simulink model "proyecto_simulink"  (R2023b)
settings: Solver=VariableStepAuto  StartTime=0.0  StopTime=0.1  RelTol=1e-3
undefined symbols (not defined in the file): test_ac1, test_ac2, test_ac3, test_am1, test_am2, test_am3, test_fc1, test_fc1_receptor, test_fc2, test_fc2_receptor, test_fc3, test_fc3_receptor, test_fm1, test_fm2, test_fm3, test_mu, test_noise_factor, test_ts
libraries: commanapbnd3 x4
settings Model: Creator=RomaW11  LastModifiedBy=RomaW11

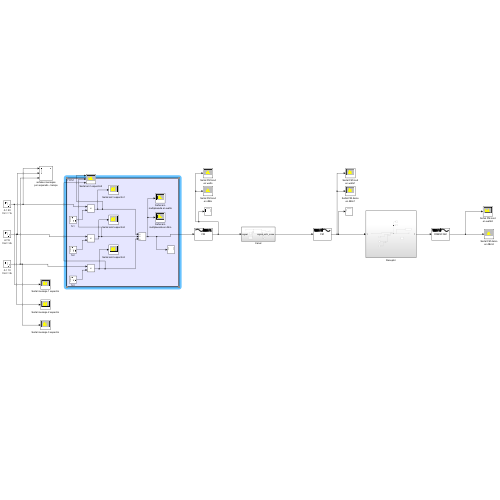
[thumbnail: Simulink's stored preview of the top-level diagram]
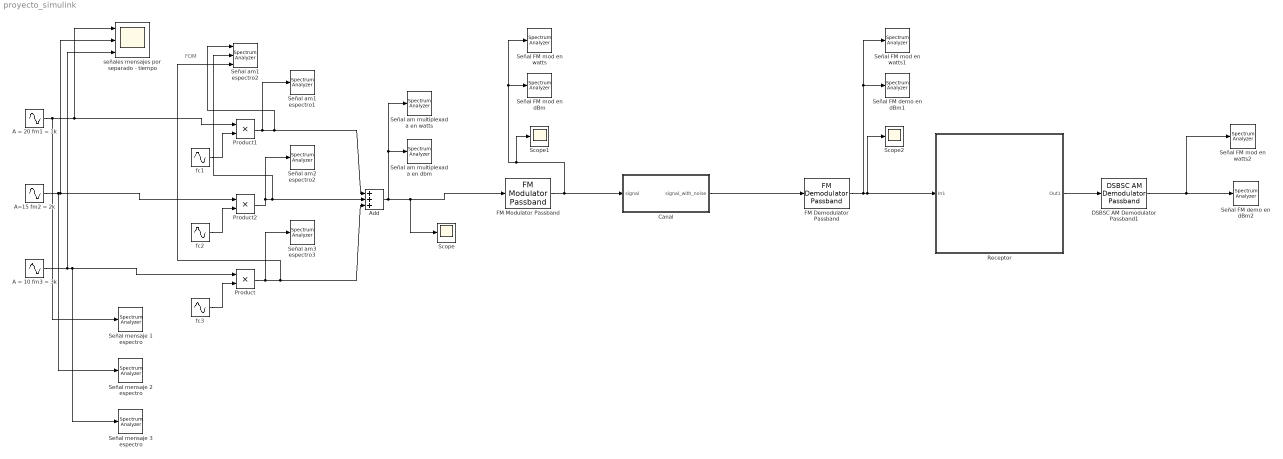
== system proyecto_simulink ==
  note: FDM
  A = 10 fm3 = 3k : Sin  Amplitude=test_am3  Frequency=2*pi*test_fm3  Phase=pi/2  SampleTime=test_ts
  A = 20 fm1 = 1k : Sin  Amplitude=test_am1  Frequency=2*pi*test_fm1  SampleTime=test_ts
  A=15 fm2 = 2k : Sin  Amplitude=test_am2  Frequency=2*pi*test_fm2  Phase=pi/2  SampleTime=test_ts
  Add : Sum  Inputs=+++
  Canal : Subsystem
  DSBSC AM Demodulator Passband1 : commanapbnd3/DSBSC AM Demodulator Passband  Fc=test_FI  Ph=0  method=Butterworth  n=4  cf=5e3  Rp=0.1  Rs=50
  FM Demodulator Passband : commanapbnd3/FM Demodulator Passband  Fc=test_FM_mod  Ph=0  Kc=50  Ho=100
  FM Modulator Passband : commanapbnd3/FM Modulator Passband  Fc=test_FM_mod  Ph=0  Kc=50
  Product : Product
  Product1 : Product
  Product2 : Product
  Receptor : Subsystem
  Scope : Scope
  Scope1 : Scope
  Scope2 : Scope
  Señal FM demo en dBm1 : SpectrumAnalyzer  WindowPosition=[1.000000,1.000000,1920.000000,1057.000000,]  ScopeFrameLocation=window  SampleRate=44.1e3  StartFrequency=20  StopFrequency=20e3  YLimits=[-84.49489701,58.22565386]  ShowLegend=on  SelectedToolstripTab=spectrumAnalyzerToolstrip.spectrumTab
      settings: OpenAtSimulationStart=off
  Señal FM demo en dBm2 : SpectrumAnalyzer  WindowPosition=[1.000000,1.000000,1920.000000,1057.000000,]  ScopeFrameLocation=window  SampleRate=44.1e3  StartFrequency=20  StopFrequency=20e3  YLimits=[-268.52169579,72.08888047]  ShowLegend=on  SelectedToolstripTab=spectrumAnalyzerToolstrip.spectrumTab
      settings: OpenAtSimulationStart=off
  Señal FM mod en dBm : SpectrumAnalyzer  WindowPosition=[1.000000,1.000000,1920.000000,1057.000000,]  ScopeFrameLocation=window  SampleRate=44.1e3  StartFrequency=20  StopFrequency=20e3  YLimits=[-251.7836109,52.91268426]  ShowLegend=on  SelectedToolstripTab=spectrumAnalyzerToolstrip.spectrumTab
      settings: OpenAtSimulationStart=off
  Señal FM mod en watts : SpectrumAnalyzer  WindowPosition=[1.000000,1.000000,1920.000000,1057.000000,]  ScopeFrameLocation=window  SampleRate=44.1e3  StartFrequency=20  StopFrequency=20e3  SpectrumUnits=Watts  YLimits=[-0.02193893,0.19745039]  ShowLegend=on  SelectedToolstripTab=spectrumAnalyzerToolstrip.spectrumTab
      settings: OpenAtSimulationStart=off
  Señal FM mod en watts1 : SpectrumAnalyzer  WindowPosition=[1.000000,1.000000,1920.000000,1057.000000,]  ScopeFrameLocation=window  SampleRate=44.1e3  StartFrequency=20  StopFrequency=20e3  SpectrumUnits=Watts  YLimits=[-3.1064895,27.95840554]  ShowLegend=on  SelectedToolstripTab=spectrumAnalyzerToolstrip.spectrumTab
      settings: OpenAtSimulationStart=off
  Señal FM mod en watts2 : SpectrumAnalyzer  WindowPosition=[1.000000,1.000000,1920.000000,1057.000000,]  ScopeFrameLocation=window  SampleRate=44.1e3  StartFrequency=20  StopFrequency=20e3  SpectrumUnits=Watts  YLimits=[-0.75147585,6.76328261]  ShowLegend=on  SelectedToolstripTab=spectrumAnalyzerToolstrip.spectrumTab
      settings: OpenAtSimulationStart=off
  Señal am multiplexada en dbm : SpectrumAnalyzer  WindowPosition=[1.000000,1.000000,1920.000000,1057.000000,]  ScopeFrameLocation=window  SampleRate=44.1e3  StartFrequency=20  StopFrequency=20e3  YLimits=[-77.52245995,57.44981241]  ShowLegend=on  SelectedToolstripTab=spectrumAnalyzerToolstrip.spectrumTab
      settings: OpenAtSimulationStart=off
  Señal am multiplexada en watts : SpectrumAnalyzer  WindowPosition=[1.000000,1.000000,1920.000000,1057.000000,]  ScopeFrameLocation=window  SampleRate=44.1e3  StartFrequency=20  StopFrequency=20e3  SpectrumUnits=Watts  YLimits=[-3.10576456,27.95188106]  ShowLegend=on  SelectedToolstripTab=spectrumAnalyzerToolstrip.spectrumTab
      settings: OpenAtSimulationStart=off
  Señal am1 espectro1 : SpectrumAnalyzer  WindowPosition=[1.000000,1.000000,1920.000000,1057.000000,]  ScopeFrameLocation=window  SampleRate=44.1e3  StartFrequency=20  StopFrequency=20e3  SpectrumUnits=Watts  YLimits=[-3.10576466,27.9518819]  ShowLegend=on  SelectedToolstripTab=spectrumAnalyzerToolstrip.spectrumTab
      settings: OpenAtSimulationStart=off
  Señal am1 espectro2 : SpectrumAnalyzer  NumInputPorts=3  WindowPosition=[1.000000,1.000000,1920.000000,1057.000000,]  ScopeFrameLocation=window  SampleRate=44.1e3  StartFrequency=20  StopFrequency=20e3  SpectrumUnits=Watts  YLimits=[-3.10576466,27.9518819]  ShowLegend=on
      settings: OpenAtSimulationStart=off
  Señal am2 espectro2 : SpectrumAnalyzer  WindowPosition=[1.000000,1.000000,1920.000000,1057.000000,]  ScopeFrameLocation=window  SampleRate=44.1e3  StartFrequency=20  StopFrequency=20e3  SpectrumUnits=Watts  YLimits=[-1.72478242,15.52304178]  ShowLegend=on  SelectedToolstripTab=spectrumAnalyzerToolstrip.spectrumTab
      settings: OpenAtSimulationStart=off
  Señal am3 espectro3 : SpectrumAnalyzer  WindowPosition=[1.000000,1.000000,1920.000000,1057.000000,]  ScopeFrameLocation=window  SampleRate=44.1e3  StartFrequency=20  StopFrequency=20e3  SpectrumUnits=Watts  YLimits=[-0.78111251,7.03001259]  ShowLegend=on  SelectedToolstripTab=spectrumAnalyzerToolstrip.spectrumTab
      settings: OpenAtSimulationStart=off
  Señal mensaje 1 espectro : SpectrumAnalyzer  WindowPosition=[1.000000,1.000000,1920.000000,1057.000000,]  ScopeFrameLocation=window  SampleRate=44.1e3  StartFrequency=20  StopFrequency=20e3  SpectrumUnits=Watts  YLimits=[-12.49984028,112.49856251]  ShowLegend=on  SelectedToolstripTab=spectrumAnalyzerToolstrip.spectrumTab
      settings: OpenAtSimulationStart=off
  Señal mensaje 2 espectro : SpectrumAnalyzer  WindowPosition=[1.000000,1.000000,1920.000000,1057.000000,]  ScopeFrameLocation=window  SampleRate=44.1e3  StartFrequency=20  StopFrequency=20e3  SpectrumUnits=Watts  YLimits=[-7.03105985,63.27953861]  ShowLegend=on  SelectedToolstripTab=spectrumAnalyzerToolstrip.spectrumTab
      settings: OpenAtSimulationStart=off
  Señal mensaje 3 espectro : SpectrumAnalyzer  WindowPosition=[1.000000,1.000000,1920.000000,1057.000000,]  ScopeFrameLocation=window  SampleRate=44.1e3  StartFrequency=20  StopFrequency=20e3  SpectrumUnits=Watts  YLimits=[-3.12012674,28.08114066]  ShowLegend=on  SelectedToolstripTab=spectrumAnalyzerToolstrip.spectrumTab
      settings: OpenAtSimulationStart=off
  fc1 : Sin  Amplitude=test_ac1  Frequency=2*pi*test_fc1  SampleTime=test_ts  VectorParams1D=off
  fc2 : Sin  Amplitude=test_ac2  Frequency=2*pi*test_fc2  Phase=pi/2  SampleTime=test_ts
  fc3 : Sin  Amplitude=test_ac3  Frequency=2*pi*test_fc3  Phase=pi/2  SampleTime=test_ts
  señales mensajes por separado - tiempo : Scope  NumInputPorts=3
  wires:
  Add/1 -> FM Modulator Passband/1, Scope/1, Señal am multiplexada en dbm/1, Señal am multiplexada en watts/1
  FM Demodulator Passband/1 -> Scope2/1, Receptor/1(In1), Señal FM mod en watts1/1, Señal FM demo en dBm1/1
  Receptor/1(Out1) -> DSBSC AM Demodulator Passband1/1
  FM Modulator Passband/1 -> Señal FM mod en watts/1, Señal FM mod en dBm/1, Scope1/1, Canal/1(signal)
  DSBSC AM Demodulator Passband1/1 -> Señal FM mod en watts2/1, Señal FM demo en dBm2/1
  Canal/1(signal_with_noise) -> FM Demodulator Passband/1
  A=15 fm2 = 2k/1 -> Product2/1, señales mensajes por separado - tiempo/2, Señal mensaje 2 espectro/1
  A = 10 fm3 = 3k/1 -> Product/1, Señal mensaje 3 espectro/1, señales mensajes por separado - tiempo/3
  fc3/1 -> Product/2
  Product1/1 -> Señal am1 espectro2/1, Add/1, Señal am1 espectro1/1
  Product/1 -> Señal am3 espectro3/1, Señal am1 espectro2/3, Add/3
  Product2/1 -> Señal am2 espectro2/1, Señal am1 espectro2/2, Add/2
  fc2/1 -> Product2/2
  fc1/1 -> Product1/2
  A = 20 fm1 = 1k/1 -> Product1/1, señales mensajes por separado - tiempo/1, Señal mensaje 1 espectro/1

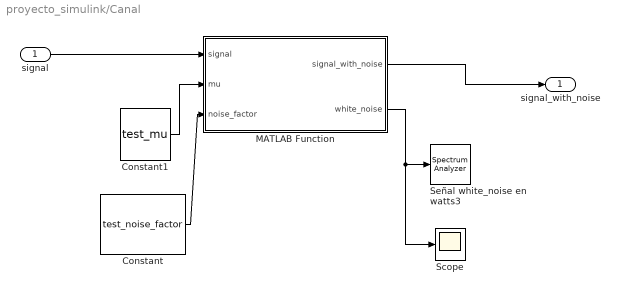
== system proyecto_simulink/Canal ==
  signal : Inport
  Constant : Constant  Value=test_noise_factor  SampleTime=test_ts
  Constant1 : Constant  Value=test_mu
  MATLAB Function : MATLAB Function  TreatAsAtomicUnit=on
  Scope : Scope
  Señal white_noise en watts3 : SpectrumAnalyzer  WindowPosition=[1.000000,1.000000,1920.000000,1057.000000,]  ScopeFrameLocation=window  SampleRate=44.1e3  StartFrequency=20  StopFrequency=20e3  YLimits=[-3603.44492261,-2802.67938425]  ShowLegend=on  SelectedToolstripTab=spectrumAnalyzerToolstrip.spectrumTab
      settings: OpenAtSimulationStart=off
  signal_with_noise : Outport
  wires:
  MATLAB Function/2(white_noise) -> Scope/1, Señal white_noise en watts3/1
  MATLAB Function/1(signal_with_noise) -> signal_with_noise/1
  Constant/1 -> MATLAB Function/3(noise_factor)
  Constant1/1 -> MATLAB Function/2(mu)
  signal/1 -> MATLAB Function/1(signal)

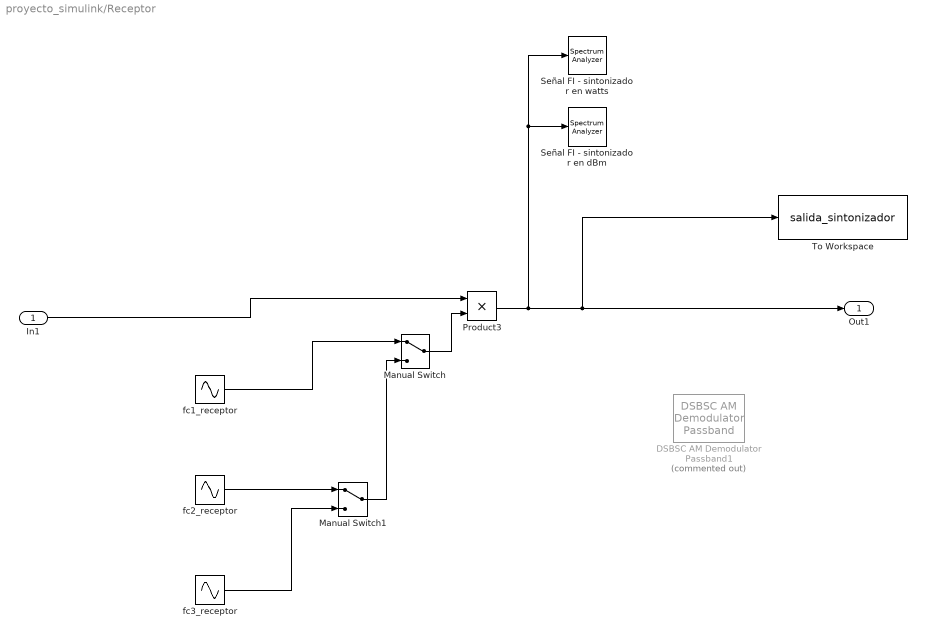
== system proyecto_simulink/Receptor ==
  In1 : Inport
  DSBSC AM Demodulator Passband1 : commanapbnd3/DSBSC AM Demodulator Passband  Commented=on  Fc=test_FI  Ph=0  method=Butterworth  n=4  cf=5e3  Rp=0.1  Rs=50
  Manual Switch : ManualSwitch
  Manual Switch1 : ManualSwitch
  Product3 : Product
  Señal FI - sintonizador en dBm : SpectrumAnalyzer  WindowPosition=[1.000000,1.000000,1920.000000,1057.000000,]  ScopeFrameLocation=window  SampleRate=44.1e3  StartFrequency=20  StopFrequency=20e3  YLimits=[-183.2628892,62.54011418]  ShowLegend=on  SelectedToolstripTab=spectrumAnalyzerToolstrip.spectrumTab
      settings: OpenAtSimulationStart=off
  Señal FI - sintonizador en watts : SpectrumAnalyzer  WindowPosition=[1.000000,1.000000,1920.000000,1057.000000,]  ScopeFrameLocation=window  SampleRate=44.1e3  StartFrequency=20  StopFrequency=20e3  SpectrumUnits=Watts  YLimits=[-0.78143237,7.03289133]  ShowLegend=on  SelectedToolstripTab=spectrumAnalyzerToolstrip.spectrumTab
      settings: OpenAtSimulationStart=off
  To Workspace : ToWorkspace  VariableName=salida_sintonizador  SampleTime=test_ts
      settings: Save2DSignal=2-D array (concatenate along first dimension)
  fc1_receptor : Sin  Frequency=2*pi*test_fc1_receptor  SampleTime=test_ts  VectorParams1D=off
  fc2_receptor : Sin  Frequency=2*pi*test_fc2_receptor  SampleTime=test_ts  VectorParams1D=off
  fc3_receptor : Sin  Frequency=2*pi*test_fc3_receptor  SampleTime=test_ts  VectorParams1D=off
  Out1 : Outport
  wires:
  Manual Switch/1 -> Product3/2
  Product3/1 -> Out1/1, To Workspace/1, Señal FI - sintonizador en watts/1, Señal FI - sintonizador en dBm/1
  Manual Switch1/1 -> Manual Switch/2
  fc2_receptor/1 -> Manual Switch1/1
  In1/1 -> Product3/1
  fc3_receptor/1 -> Manual Switch1/2
  fc1_receptor/1 -> Manual Switch/1

== matlab function proyecto_simulink/Canal/MATLAB Function ==
  data: signal input; signal_with_noise output; white_noise output; mu input; noise_factor input
function [signal_with_noise, white_noise] = awgn_noise(signal, mu, noise_factor)
    % WHITE_NOISE Genera ruido blanco basado en la señal de entrada.
    %
    % Inputs:
    %   signal - Señal de entrada (vector).
    %
    % Outputs:
    %   white_noise - Vector de ruido blanco generado.
    
    % Media del ruido
    % mu = 0;
    
    % Desviación estándar proporcional a la señal de entrada
    sigma = noise_factor * std(signal);
    
    % Generar ruido blanco (distribución normal)
    white_noise = mu + sigma * randn(size(signal));
    signal_with_noise = signal + white_noise;
end
